simulink model "a4fallschirmSim_lsg"  (R2018b)
settings: Solver=VariableStepAuto  StartTime=0.0  StopTime=inf  RelTol=1e-3  EnableMultiTasking=on
StopFcn:
  | ergDisc=[tout yout];
  | clear tout;
  | clear yout;
model workspace (MAT data in the model file):
  AFS = 30
  AS = 0.5
  DT = 2
  cw = 1.3
  g = 9.81
  h0 = 300
  h1 = 200
  m = 85
  rho = 1.2
  v0 = 0
settings Model: Creator=Reichl  LastModifiedBy=Reichl
settings DataIOCC: SaveFormat=Array
settings OptimizationCC: LifeSpan=inf
settings DebuggingCC: SolverPrmCheckMsg=warning  AllowSymbolicDim=off  SFUnexpectedBacktrackingDiag=warning  SFNoUnconditionalDefaultTransitionDiag=warning  SFExecutionAtInitializationDiag=none
settings HardwareCC: ProdBitPerPointer=32  ProdBitPerSizeT=32  ProdBitPerPtrDiffT=32  ProdLargestAtomicFloat=None  ProdIntDivRoundTo=Undefined  ProdEndianess=Unspecified  ProdWordSize=32  ProdHWDeviceType=32-bit Generic
settings ModelReferenceCC: PropagateSignalLabelsOutOfModel=off
settings SFSimCC: SimUseLocalCustomCode=off
settings RTWCC: RTWUseLocalCustomCode=off
settings CodeAppCC: StateflowObjectComments=on
settings GRTTargetCC: TargetLangStandard=C89/C90 (ANSI)  GeneratePreprocessorConditionals=Disable all
settings ConfigComp: CovMetricSettings=dw  CovHtmlReporting=on  CovSaveCumulativeToWorkspaceVar=on  CovSaveSingleToWorkspaceVar=on  CovExternalEMLEnable=off  CovSFcnEnable=off

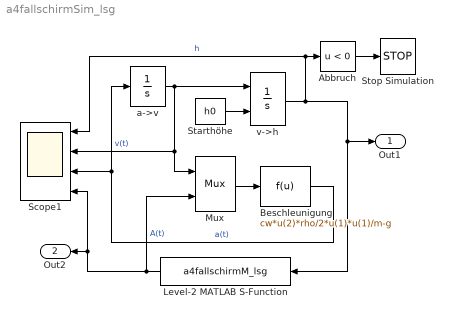
== system a4fallschirmSim_lsg ==
  Abbruch : Fcn  Expr=u < 0
  Beschleunigung : Fcn  Expr=cw*u(2)*rho/2*u(1)*u(1)/m-g
  Level-2 MATLAB S-Function : M-S-Function  FunctionName=a4fallschirmM_lsg  Parameters="AS AFS h1  DT"
  Mux : Mux  Inputs=2
      settings: DisplayOption=signals
  Scope1 : Scope  NumInputPorts=4
  Starthöhe : Constant  Value=h0
  Stop Simulation : Stop
  a->v : Integrator  InitialCondition=v0
  v->h : Integrator  InitialConditionSource=external
  Out1 : Outport
  Out2 : Outport  Port=2
  wires:
  a->v/1 -> Scope1/2, Mux/1, v->h/1  "v(t)"
  v->h/1 -> Out1/1, Level-2 MATLAB S-Function/1, Scope1/1, Abbruch/1  "h"
  Abbruch/1 -> Stop Simulation/1
  Starthöhe/1 -> v->h/2
  Mux/1 -> Beschleunigung/1
  Beschleunigung/1 -> a->v/1, Scope1/3  "a(t)"
  Level-2 MATLAB S-Function/1 -> Mux/2, Out2/1, Scope1/4  "A(t)"
